simulink model "admire_sim_NDI"  (Simulink 8.4)
settings: Solver=ode4  SolverMode=SingleTasking  StartTime=0.0  StopTime=1000  FixedStep=dt  RelTol=1e-3  AbsTol=1e-6
InitFcn:
  | INIT_NDI
StartFcn:
  | tic
StopFcn:
  | toctime=toc;
  | fprintf('Actual Time = %g\nSim Time = %g\n',toctime,tout(end))
  | % Make plots
  | %admire_sim_plot
  | figure
  | plot3(yout(:,11),yout(:,10),-yout(:,12),'*-');grid
  | xlabel('East (m)');ylabel('North (m)');zlabel('Alt (m)')
  | view([0 0 1])
  | hold on
  | plot3(Ywpt,Xwpt,0*Xwpt,'r^-','MarkerSize',10)
  | axis equal
  | hold off
values from neighbouring files (symbols this model uses):
  a1 = (180*d2r)/(80^3)    (= 6.13592315154e-06)    [INIT_LINEAR.m]    (also in INIT_NDI.m)
  a2 = (24*d2r)/(80^3)    (= 8.18123086872e-07)    [INIT_LINEAR.m]    (also in INIT_NDI.m)
  Abare = [-0.0369710265542 -0.00338320638614 0 0 0.00101076287488 0 0 0 0 1.00000000002 0 1.7763568394e-12 ... (784 elements, 28x28)]    [Trim_M0p22ALT20_LinDATA.mat]    (also in Trim_M0p3ALT2000_LinDATA.mat = [-0.0208061645292 -0.00191640084378 0 0 0.000610808752105 0 )
  Altcmd_t = [ 0    1   100 200  300  425  450  550  600  700  800  880  980]    [INIT_NDI.m]
  Altcmd_v = [20  20   20   1500 1500 1500 1500 3000 3000 4000 4000 6000 6000]    [INIT_NDI.m]
  Bbare = [-1.10043807057 0.00182125944543 -0.00701366565749 0.707306131876 1.12037014439 -0.330899025785 0 0 0 0 0 0 ... (448 elements, 28x16)]    [Trim_M0p22ALT20_LinDATA.mat]    (also in Trim_M0p3ALT2000_LinDATA.mat = [-1.42042676365 -0.000549876720984 -0.00633411409606 0.84954)
  bref = 10    [INIT_NDI.m]
  C1 = ((Iy-Iz)*Iz-Ixz^2)/GG    (= -0.958151081688)    [INIT_NDI.m]
  C2 = (Ix-Iy+Iz)*Ixz/GG    (= 0.0484690861804)    [INIT_NDI.m]
  C3 = Iz/GG    (= 4.77597824802e-05)    [INIT_NDI.m]
  C4 = Ixz/GG    (= 1.18217283367e-06)    [INIT_NDI.m]
  C5 = (Iz-Ix)/Iy    (= 0.987654320988)    [INIT_NDI.m]
  C6 = Ixz/Iy    (= 0.0308641975309)    [INIT_NDI.m]
  C7 = 1/Iy    (= 1.23456790123e-05)    [INIT_NDI.m]
  C8 = (Ix*(Ix-Iy)+Ixz^2)/GG    (= -0.592859676085)    [INIT_NDI.m]
  C9 = Ix/GG    (= 9.93025180281e-06)    [INIT_NDI.m]
  CAmethod = 1    [ACA_init.m]    (also in INIT_LINEAR.m = 0; INIT_NDI.m = 0)
  Canard_max = interp1(M_vec,[25 25 25 15 15 15 15 15]*d2r,Mach,'next')    [INIT_LINEAR.m]    (also in INIT_NDI.m = [25 25 25 15 15 15 15 15]*d2r)
  Canard_min = interp1(M_vec,[-55 -55 -25 -15 -15 -15 -15 -15]*d2r,Mach,'next')    [INIT_LINEAR.m]    (also in INIT_NDI.m = [-55 -55 -25 -15 -15 -15 -15 -15]*d2r)
  CB = zeros(3,NumU)    [ACA_init.m]    (also in INIT_NDI.m = CCV*Bbare)
  CC = [C3 0 C4;0 C7 0;C4 0 C9]    [INIT_NDI.m]
  CCV = [CCV zeros(3,22)]    [INIT_LINEAR.m]    (also in INIT_NDI.m)
  cref = 5.2    [INIT_NDI.m]
  d2r = pi/180    (= 0.0174532925199)    [ACA_init.m]    (also in INIT_LINEAR.m; INIT_NDI.m)
  dalpha_err = 0    [Trim_M0p22ALT20_LinDATA.mat]    (also in Trim_M0p3ALT2000_LinDATA.mat)
  dalt_err = 0    [Trim_M0p22ALT20_LinDATA.mat]    (also in Trim_M0p3ALT2000_LinDATA.mat)
  dbeta_err = 0    [Trim_M0p22ALT20_LinDATA.mat]    (also in Trim_M0p3ALT2000_LinDATA.mat)
  ddc_bw = 0    [Trim_M0p22ALT20_LinDATA.mat]    (also in Trim_M0p3ALT2000_LinDATA.mat)
  ddc_rate = 0    [Trim_M0p22ALT20_LinDATA.mat]    (also in Trim_M0p3ALT2000_LinDATA.mat)
  ddei_bw = 0    [Trim_M0p22ALT20_LinDATA.mat]    (also in Trim_M0p3ALT2000_LinDATA.mat)
  ddei_rate = 0    [Trim_M0p22ALT20_LinDATA.mat]    (also in Trim_M0p3ALT2000_LinDATA.mat)
  ddey_bw = 0    [Trim_M0p22ALT20_LinDATA.mat]    (also in Trim_M0p3ALT2000_LinDATA.mat)
  ddey_rate = 0    [Trim_M0p22ALT20_LinDATA.mat]    (also in Trim_M0p3ALT2000_LinDATA.mat)
  ddle_bw = 0    [Trim_M0p22ALT20_LinDATA.mat]    (also in Trim_M0p3ALT2000_LinDATA.mat)
  ddle_rate = 0    [Trim_M0p22ALT20_LinDATA.mat]    (also in Trim_M0p3ALT2000_LinDATA.mat)
  ddr_bw = 0    [Trim_M0p22ALT20_LinDATA.mat]    (also in Trim_M0p3ALT2000_LinDATA.mat)
  ddr_rate = 0    [Trim_M0p22ALT20_LinDATA.mat]    (also in Trim_M0p3ALT2000_LinDATA.mat)
  dt = 0.01    [ACA_init.m]    (also in INIT_LINEAR.m; INIT_NDI.m)
  DTY_max = 0.002    [ACA_init.m]    (also in INIT_LINEAR.m; INIT_NDI.m)
  DTY_min = -0.002    [ACA_init.m]    (also in INIT_LINEAR.m; INIT_NDI.m)
  DTZ_max = 0.002    [ACA_init.m]    (also in INIT_LINEAR.m; INIT_NDI.m)
  DTZ_min = -0.002    [ACA_init.m]    (also in INIT_LINEAR.m; INIT_NDI.m)
  du = [eye(7,7)*d2r eye(7,7)*(-d2r);zeros(20,14)]    [INIT_NDI.m]
  dVt_err = 0    [Trim_M0p22ALT20_LinDATA.mat]    (also in Trim_M0p3ALT2000_LinDATA.mat)
  dx0bare = [-0.418180446269 0.000900932997672 0 0 -2.2213523116e-08 0 0 0 0 74.8477877145 0 0]    [Trim_M0p22ALT20_LinDATA.mat]    (also in Trim_M0p3ALT2000_LinDATA.mat = [-0.342751146187 0.000400431081223 0 0 -4.49007756074e-09 0 )
  Elevon_max = interp1(M_vec,[30 30 25 25 25 25 25 25]*d2r,Mach,'next')    [INIT_LINEAR.m]    (also in INIT_NDI.m = [30 30 25 25 25 25 25 25]*d2r)
  Elevon_min = interp1(M_vec,[-30 -30 -30 -30 -30 -30 -30 -30]*d2r,Mach,'next')    [INIT_LINEAR.m]    (also in INIT_NDI.m = [-30 -30 -30 -30 -30 -30 -30 -30]*d2r)
  G = [ 0 1 0 ... (first row only)    [ACA_init.m]    (also in INIT_LINEAR.m = [ 1 0 0; INIT_NDI.m)
  kcb = 2.5    [INIT_NDI.m]
  kfb = -0.4    [INIT_NDI.m]
  kib = 0.2    [INIT_NDI.m]
  kpb = 0.8    [INIT_NDI.m]
  LEF_max = interp1(M_vec,[30 30 30 20 20 15 10 10]*d2r,Mach,'next')    [INIT_LINEAR.m]    (also in INIT_NDI.m = [30 30 30 20 20 15 10 10]*d2r)
  LEF_min = interp1(M_vec,[-10 -10 -10 -10 -10 -10 -10 -10]*d2r,Mach,'next')    [INIT_LINEAR.m]    (also in INIT_NDI.m = [-10 -10 -10 -10 -10 -10 -10 -10]*d2r)
  LG_max = 1    [ACA_init.m]    (also in INIT_LINEAR.m; INIT_NDI.m)
  LG_min = 0    [ACA_init.m]    (also in INIT_LINEAR.m; INIT_NDI.m)
  LPmethod = 3    [ACA_init.m]    (also in INIT_LINEAR.m = 0; INIT_NDI.m = 0; LPwrap.m = 0; LPwrap_1.m = 0)
  M_vec = [0 0 0]    [DAwrap.m]    (also in INIT_LINEAR.m = [0 0.5 0.8 0.9 0.95 1.4 1.5 2.5]; INIT_NDI.m = [0 0.5 0.8 0.9 0.95 1.4 1.5 2.5])
  mass = 9100    [INIT_NDI.m]
  NumU = 16    [ACA_init.m]    (also in INIT_LINEAR.m; INIT_NDI.m; test.m; test_LPwrap.m)
  nwpt = 5    [INIT_NDI.m]
  PD_max = 10    [ACA_init.m]    (also in INIT_LINEAR.m; INIT_NDI.m)
  PD_min = -10    [ACA_init.m]    (also in INIT_LINEAR.m; INIT_NDI.m)
  PHIcmd_t = [0 1 1+dt 30 30+dt 60 60+dt 90 90+dt 120 120+dt 150 150+dt 180 180+dt 210 210+dt 240 240+dt 270 270+dt 300 300+dt 330 330+dt]    [INIT_NDI.m]
  PHIcmd_v = [0 0 15   15 -15   -15 0    0   30   30  -30    -30 0      0   45     45   0     0    -45   -45   0     0   -60   -60 0]    [INIT_NDI.m]
  Pmode = 3    [INIT_NDI.m]
  r2d = 180/pi    (= 57.2957795131)    [ACA_init.m]    (also in INIT_LINEAR.m; INIT_NDI.m)
  rlimit_c = 0.87260034904    [Trim_M0p22ALT20_LinDATA.mat]    (also in Trim_M0p3ALT2000_LinDATA.mat)
  rlimit_ie = 2.61780104712    [Trim_M0p22ALT20_LinDATA.mat]    (also in Trim_M0p3ALT2000_LinDATA.mat)
  rlimit_le = 0.174520069808    [Trim_M0p22ALT20_LinDATA.mat]    (also in Trim_M0p3ALT2000_LinDATA.mat)
  rlimit_oe = 2.61780104712    [Trim_M0p22ALT20_LinDATA.mat]    (also in Trim_M0p3ALT2000_LinDATA.mat)
  rlimit_r = 1.74520069808    [Trim_M0p22ALT20_LinDATA.mat]    (also in Trim_M0p3ALT2000_LinDATA.mat)
  Rmode = 3    [INIT_NDI.m]
  Rudder_max = interp1(M_vec,[30 30 25 20 15 15 15 10]*d2r,Mach,'next')    [INIT_LINEAR.m]    (also in INIT_NDI.m = [30 30 25 20 15 15 15 10]*d2r)
  Rudder_min = interp1(M_vec,[-30 -30 -25 -20 -15 -15 -15 -10]*d2r,Mach,'next')    [INIT_LINEAR.m]    (also in INIT_NDI.m = [-30 -30 -25 -20 -15 -15 -15 -10]*d2r)
  Sref = 45    [INIT_NDI.m]
  TSS_max = 1    [ACA_init.m]    (also in INIT_LINEAR.m; INIT_NDI.m)
  TSS_min = 0    [ACA_init.m]    (also in INIT_LINEAR.m; INIT_NDI.m)
  u0fcs = [0 74.8477877145 0 0 -0.0114511280235]    [Trim_M0p22ALT20_LinDATA.mat]    (also in Trim_M0p3ALT2000_LinDATA.mat = [0 99.7587452043 0 0 -0.00434812413209])
  u0new = [-0.00172441963734 -0.00172441963734 0.0557681770547 0.0557681770547 0.0557681770547 0.0557681770547 0 0 0 0.0785 0 0 ... (16 elements, 16x1)]    [Trim_M0p22ALT20_LinDATA.mat]    (also in Trim_M0p3ALT2000_LinDATA.mat = [-0.00056590748572 -0.00056590748572 0.0273345559009 0.02733)
  UD_max = 10    [ACA_init.m]    (also in INIT_LINEAR.m; INIT_NDI.m)
  UD_min = -10    [ACA_init.m]    (also in INIT_LINEAR.m; INIT_NDI.m)
  Upref = [0 0 0 0 0 0 0 0 0 0 0 0 0 0 0 0]'    [ACA_init.m]    (also in INIT_LINEAR.m; INIT_NDI.m)
  Upref_split = [[0 0 30 -30 -30 30 0]*d2r*.4 0 0 0 0 0 0 0 0 0]'    [INIT_NDI.m]
  Urlim = [350*d2r ... (first row only)    [ACA_init.m]    (also in INIT_NDI.m = [50*d2r)
  UseRL = 0    [ACA_init.m]    (also in INIT_NDI.m)
  Vcmd_t = [  0    1   100  200  300  425  450  550  600  700  800  880  980]    [INIT_NDI.m]
  Vcmd_v = Mcmd_v.*a    [INIT_NDI.m]
  VD_max = 10    [ACA_init.m]    (also in INIT_LINEAR.m; INIT_NDI.m)
  VD_min = -10    [ACA_init.m]    (also in INIT_LINEAR.m; INIT_NDI.m)
  WD_max = 10    [ACA_init.m]    (also in INIT_LINEAR.m; INIT_NDI.m)
  WD_min = -10    [ACA_init.m]    (also in INIT_LINEAR.m; INIT_NDI.m)
  Wp = W'*W    [ACA_init.m]    (also in INIT_LINEAR.m; INIT_NDI.m; test.m; test_LPwrap.m)
  Wpts = [0 1 2 3 4]    [INIT_NDI.m]
  x0 = [ max(eyp,zeros(n,1));max(-eyp,zeros(n,1));zeros(2*m,1)]    [LPwrap.m]    (also in LPwrap_1.m; LPwrap_par.m; Trim_M0p22ALT20_LinDATA.mat = [-8.62209818672e-05 -8.62209818672e-05 0.00278840885273 0.00; Trim_M0p3ALT2000_LinDATA.mat = [-2.8295374286e-05 -2.8295374286e-05 0.00136672779504 0.0013)
  x0bare = [74.8477877145 0.159877852888 0 0 0 0 0 0.159877852888 0 0 0 -20]    [Trim_M0p22ALT20_LinDATA.mat]    (also in Trim_M0p3ALT2000_LinDATA.mat = [99.7587452043 0.116024082006 0 0 0 0 0 0.116024082006 0 0 0)
  Xwpt = [0 4000 4000 0 0]*8    [INIT_NDI.m]
  y0bare = [74.8477877145 0.159877852888 0 0 0 0 0 0.159877852888 0 0 0 -20 ... (73 elements, 73x1)]    [Trim_M0p22ALT20_LinDATA.mat]    (also in Trim_M0p3ALT2000_LinDATA.mat = [99.7587452043 0.116024082006 0 0 0 0 0 0.116024082006 0 0 0)
  Ywpt = [0 0 4000 4000 0]*8    [INIT_NDI.m]
undefined symbols (not defined in the file or in its folder): CGIwrap, DAwrap, LPwrap, VJAwrap
libraries: simulink_extras x19, simulink x12
(part 5 of 5)

== system admire_sim_NDI/NDI_CLAW/DynamicInversionControl/ControlAllocation/GetU/WeightedPseudo Scaled_2/Blocks/Some_Saturated/For Iterator Subsystem/If Action Subsystem1/If Action Subsystem1 ==
  Action Port : ActionPort  ActionType=else
  Constant4 : Constant  Value=0
  Out1 : Outport
  wires:
  Constant4/1 -> Out1/1

== system admire_sim_NDI/NDI_CLAW/DynamicInversionControl/ControlAllocation/GetU/WeightedPseudo Scaled_2/Blocks/Some_Saturated/For Iterator Subsystem/If Action Subsystem2/If Action Subsystem ==
  u : Inport
  ulim : Inport  Port=2
  scale_z : Inport  Port=3
  Action Port : ActionPort  ActionType=then
  MinMax : MinMax  Inputs=2
  Product : Product  Inputs=*/  RndMeth=Zero
  Out1 : Outport
  wires:
  MinMax/1 -> Out1/1
  Product/1 -> MinMax/1
  u/1 -> Product/2
  ulim/1 -> Product/1
  scale_z/1 -> MinMax/2

== system admire_sim_NDI/NDI_CLAW/DynamicInversionControl/ControlAllocation/GetU/WeightedPseudo Scaled_2/Blocks/Some_Saturated/For Iterator Subsystem/If Action Subsystem2/If Action Subsystem1 ==
  Action Port : ActionPort  ActionType=else
  Constant4 : Constant  Value=0
  Out1 : Outport
  wires:
  Constant4/1 -> Out1/1
